simulink model "Ford_T3T6_ArchCnctnDigrm"  (R2016b)
settings: Solver=FixedStepDiscrete  StartTime=0.0  StopTime=10.0  RelTol=1e-3  EnableMultiTasking=on
libraries: canmsglib x15
(part 2 of 15)

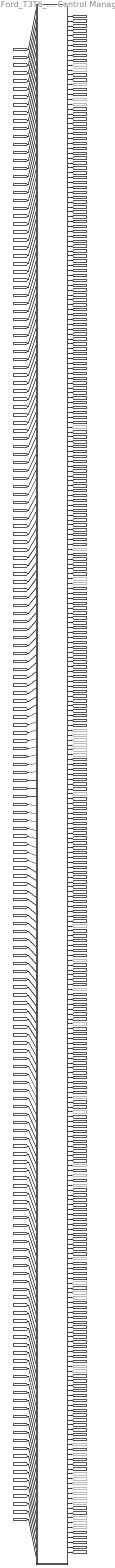
== system Ford_T3T6_ArchCnctnDigrm/Motor Control Manager ==
  AR300FORDA_MotCtrlMgr : Subsystem  Tag=1.0.X  Description=This component handles runnable scheduling of MotorControl and MotorControlx2 runnables. This also defines all of the Motor Control related data and is resposible for the runnables providing the data interface to the RTE.
      settings: AttributesFormatString=Version: %<Tag>
  AR300FORDA_MotCtrlMgr_BattRtnCurrAdc : Goto  Commented=on  GotoTag=BattRtnCurrAdc  TagVisibility=global
  AR300FORDA_MotCtrlMgr_BattRtnCurrAdcFaild : Goto  Commented=on  GotoTag=BattRtnCurrAdcFaild  TagVisibility=global
  AR300FORDA_MotCtrlMgr_BattVltgAdcFaild : Goto  Commented=on  GotoTag=BattVltgAdcFaild  TagVisibility=global
  AR300FORDA_MotCtrlMgr_CurrMeasWrmIninTestCmpl : Goto  Commented=on  GotoTag=CurrMeasWrmIninTestCmpl  TagVisibility=global
  AR300FORDA_MotCtrlMgr_EcuId : Goto  Commented=on  GotoTag=EcuId  TagVisibility=global
  AR300FORDA_MotCtrlMgr_MotBackEmfVltg : Goto  Commented=on  GotoTag=MotBackEmfVltg  TagVisibility=global
  AR300FORDA_MotCtrlMgr_MotCtrlAdc0RawRes : Goto  Commented=on  GotoTag=MotCtrlAdc0RawRes  TagVisibility=global
  AR300FORDA_MotCtrlMgr_MotCtrlAdc0ScanGroup2Ref0 : Goto  Commented=on  GotoTag=MotCtrlAdc0ScanGroup2Ref0  TagVisibility=global
  AR300FORDA_MotCtrlMgr_MotCtrlAdc0ScanGroup2Ref1 : Goto  Commented=on  GotoTag=MotCtrlAdc0ScanGroup2Ref1  TagVisibility=global
  AR300FORDA_MotCtrlMgr_MotCtrlAdc0ScanGroup3Ref0 : Goto  Commented=on  GotoTag=MotCtrlAdc0ScanGroup3Ref0  TagVisibility=global
  AR300FORDA_MotCtrlMgr_MotCtrlAdc0ScanGroup3Ref1 : Goto  Commented=on  GotoTag=MotCtrlAdc0ScanGroup3Ref1  TagVisibility=global
  AR300FORDA_MotCtrlMgr_MotCtrlAdc1RawRes : Goto  Commented=on  GotoTag=MotCtrlAdc1RawRes  TagVisibility=global
  AR300FORDA_MotCtrlMgr_MotCtrlCurrMeasMotAgCorrd : Goto  Commented=on  GotoTag=MotCtrlCurrMeasMotAgCorrd  TagVisibility=global
  AR300FORDA_MotCtrlMgr_MotCtrlMotAg5Cos : Goto  Commented=on  GotoTag=MotCtrlMotAg5Cos  TagVisibility=global
  AR300FORDA_MotCtrlMgr_MotCtrlMotAg5Sin : Goto  Commented=on  GotoTag=MotCtrlMotAg5Sin  TagVisibility=global
  AR300FORDA_MotCtrlMgr_MotCtrlMotAg6Cos : Goto  Commented=on  GotoTag=MotCtrlMotAg6Cos  TagVisibility=global
  AR300FORDA_MotCtrlMgr_MotCtrlMotAg6Sin : Goto  Commented=on  GotoTag=MotCtrlMotAg6Sin  TagVisibility=global
  AR300FORDA_MotCtrlMgr_MotCtrlMotAgElec : Goto  Commented=on  GotoTag=MotCtrlMotAgElec  TagVisibility=global
  AR300FORDA_MotCtrlMgr_MotCtrlMotAgMeasTi : Goto  Commented=on  GotoTag=MotCtrlMotAgMeasTi  TagVisibility=global
  AR300FORDA_MotCtrlMgr_MotCtrlMotCurrAdcVlyA : Goto  Commented=on  GotoTag=MotCtrlMotCurrAdcVlyA  TagVisibility=global
  AR300FORDA_MotCtrlMgr_MotCtrlMotCurrAdcVlyB : Goto  Commented=on  GotoTag=MotCtrlMotCurrAdcVlyB  TagVisibility=global
  AR300FORDA_MotCtrlMgr_MotCtrlMotCurrAdcVlyC : Goto  Commented=on  GotoTag=MotCtrlMotCurrAdcVlyC  TagVisibility=global
  AR300FORDA_MotCtrlMgr_MotCtrlMotCurrDax : Goto  Commented=on  GotoTag=MotCtrlMotCurrDax  TagVisibility=global
  AR300FORDA_MotCtrlMgr_MotCtrlMotCurrQax : Goto  Commented=on  GotoTag=MotCtrlMotCurrQax  TagVisibility=global
  AR300FORDA_MotCtrlMgr_MotCtrlMotCurrQaxCoggCmd : Goto  Commented=on  GotoTag=MotCtrlMotCurrQaxCoggCmd  TagVisibility=global
  AR300FORDA_MotCtrlMgr_MotCtrlMotCurrQaxRplCmd : Goto  Commented=on  GotoTag=MotCtrlMotCurrQaxRplCmd  TagVisibility=global
  AR300FORDA_MotCtrlMgr_MotCtrlMotModlnIdx : Goto  Commented=on  GotoTag=MotCtrlMotModlnIdx  TagVisibility=global
  AR300FORDA_MotCtrlMgr_MotCtrlMotPhaAdv : Goto  Commented=on  GotoTag=MotCtrlMotPhaAdv  TagVisibility=global
  AR300FORDA_MotCtrlMgr_MotCtrlMotVltgDax : Goto  Commented=on  GotoTag=MotCtrlMotVltgDax  TagVisibility=global
  AR300FORDA_MotCtrlMgr_MotCtrlMotVltgQax : Goto  Commented=on  GotoTag=MotCtrlMotVltgQax  TagVisibility=global
  AR300FORDA_MotCtrlMgr_MotCtrlPhaOnTiA : Goto  Commented=on  GotoTag=MotCtrlPhaOnTiA  TagVisibility=global
  AR300FORDA_MotCtrlMgr_MotCtrlPhaOnTiB : Goto  Commented=on  GotoTag=MotCtrlPhaOnTiB  TagVisibility=global
  AR300FORDA_MotCtrlMgr_MotCtrlPhaOnTiC : Goto  Commented=on  GotoTag=MotCtrlPhaOnTiC  TagVisibility=global
  AR300FORDA_MotCtrlMgr_MotCtrlPhaOnTiSumA : Goto  Commented=on  GotoTag=MotCtrlPhaOnTiSumA  TagVisibility=global
  AR300FORDA_MotCtrlMgr_MotCtrlPhaOnTiSumB : Goto  Commented=on  GotoTag=MotCtrlPhaOnTiSumB  TagVisibility=global
  AR300FORDA_MotCtrlMgr_MotCtrlPhaOnTiSumC : Goto  Commented=on  GotoTag=MotCtrlPhaOnTiSumC  TagVisibility=global
  AR300FORDA_MotCtrlMgr_MotCtrlPwmPerd : Goto  Commented=on  GotoTag=MotCtrlPwmPerd  TagVisibility=global
  AR300FORDA_MotCtrlMgr_MotCtrlSwCalEna : Goto  Commented=on  GotoTag=MotCtrlSwCalEna  TagVisibility=global
  AR300FORDA_MotCtrlMgr_MotCtrlSwCalModlnIdx : Goto  Commented=on  GotoTag=MotCtrlSwCalModlnIdx  TagVisibility=global
  AR300FORDA_MotCtrlMgr_MotCtrlSwCalPosnIdx : Goto  Commented=on  GotoTag=MotCtrlSwCalPosnIdx  TagVisibility=global
  AR300FORDA_MotCtrlMgr_MotCurrQlfr1 : Goto  Commented=on  GotoTag=MotCurrQlfr1  TagVisibility=global
  AR300FORDA_MotCtrlMgr_MotInduDaxEstimdIvs : Goto  Commented=on  GotoTag=MotInduDaxEstimdIvs  TagVisibility=global
  AR300FORDA_MotCtrlMgr_MotInduQaxEstimdIvs : Goto  Commented=on  GotoTag=MotInduQaxEstimdIvs  TagVisibility=global
  tag scope: Adc0DynRef=global, Adc0RawRes=global, Adc0ScanGroup2Ref0=global, Adc0ScanGroup2Ref1=global, Adc0ScanGroup3Ref0=global, Adc0ScanGroup3Ref1=global, Adc0SelfDiag0=global, Adc0SelfDiag2=global, Adc0SelfDiag4=global, Adc1RawRes=global, BattRtnCurrAmprFastLoop=global, BattVltgAdc=global, CmuOffs=global, CurrMeasMotAgCorrd=global, FastLoopCntr=global, HwTq0Idx=global, HwTq0MissErrCntr=global, HwTq0SentComSts=global, HwTq0SentData=global, HwTq2Idx=global, HwTq2MissErrCntr=global, HwTq2SentComSts=global, HwTq2SentData=global, HwTq4Buf=global, HwTq4RawAdc=global, HwTq4RawAdcFaild=global, HwTq4RawFastAdc=global, HwTq4RawFastAdcBuf=global, HwTq5Buf=global, HwTq5RawAdc=global, HwTq5RawAdcFaild=global, HwTq5RawFastAdc=global, HwTq5RawFastAdcBuf=global, HwTq8Idx=global, HwTq8MissErrCntr=global, HwTq8SentComSts=global, HwTq8SentData=global, MotAg0ErrReg=global, MotAg0Mecl=global, MotAg0MeclRollgCntr=global, MotAg0ParFltCnt=global, MotAg0RawMecl=global, MotAg0RawRes=global, MotAg0SpiMecl=global, MotAg0TurnCntrReg=global, MotAg0VltgFltCnt=global, MotAg0WarnReg=global, MotAg1ErrReg=global, MotAg1Mecl=global, MotAg1MeclRollgCntr=global, MotAg1ParFltCnt=global, MotAg1RawMecl=global, MotAg1RawRes=global, MotAg1SpiMecl=global, MotAg1TurnCntrReg=global, MotAg1VltgFltCnt=global, MotAg1WarnReg=global, MotAg3Mecl=global, MotAg4Mecl=global, MotAg5Cos=global, MotAg5MeasTi=global, MotAg5Mecl=global, MotAg5RawMecl=global, MotAg5Sin=global, MotAg6Cos=global, MotAg6MeasTi=global, MotAg6Mecl=global, MotAg6RawMecl=global, MotAg6Sin=global, MotAgBuf=global, MotAgBufIdx=global, MotAgBuf_SigOut=global, MotAgCumvAlgndMrfRev=global, MotAgCumvInid=global, MotAgElec=global, MotAgMeasTi=global, MotAgMecl=global, MotAgTiBuf=global, MotAgTiBuf_SigOut=global, MotCtrlAdcDiagcEndPtrOutp=global, MotCtrlAdcDiagcStrtPtrOutp=global, MotCtrlBattRtnCurrAdc=global, MotCtrlBrdgVltg=global, MotCtrlCtrlrTFild=global, MotCtrlCurrMeasCorrlnSts=global, MotCtrlCurrMeasLoaMtgtnEna=global, MotCtrlCurrMeasWrmIninTestCmpl=global, MotCtrlDiagcStsIvtr1Inactv=global, MotCtrlDiagcStsIvtr2Inactv=global, MotCtrlDualEcuMotCtrlMtgtnEna=global, MotCtrlEcuTFild=global, MotCtrlHwTq4Raw=global, MotCtrlHwTq4RawFastAdc=global, MotCtrlHwTq5Raw=global, MotCtrlHwTq5RawFastAdc=global, MotCtrlIvtrFetFltPha=global, MotCtrlIvtrFetFltTyp=global, MotCtrlIvtrLoaMtgtnEna=global, MotCtrlLoopCntr2MilliSec=global, MotCtrlMfgEnaSt=global, MotCtrlMotAg0ABIFaild=global, MotCtrlMotAg0Offs=global, MotCtrlMotAg0QepFaild=global, MotCtrlMotAg0RawRes=global, MotCtrlMotAg1ABIFaild=global, MotCtrlMotAg1Offs=global, MotCtrlMotAg1QepFaild=global, MotCtrlMotAg1RawRes=global, MotCtrlMotAg2Cos=global, MotCtrlMotAg2CosAdcFaild=global, MotCtrlMotAg2Sin=global, MotCtrlMotAg2SinAdcFaild=global, MotCtrlMotAg5CosAdcFaild=global, MotCtrlMotAg5CosRtAmpRecpr1=global, MotCtrlMotAg5CosRtAmpRecpr=global, MotCtrlMotAg5CosRtOffs1=global, MotCtrlMotAg5CosRtOffs=global, MotCtrlMotAg5Polarity=global, MotCtrlMotAg5SinAdcFaild=global, MotCtrlMotAg5SinRtAmpRecpr1=global, MotCtrlMotAg5SinRtAmpRecpr=global, MotCtrlMotAg5SinRtOffs1=global, MotCtrlMotAg5SinRtOffs=global, MotCtrlMotAg6CosAdcFaild=global, MotCtrlMotAg6CosRtAmpRecpr1=global, MotCtrlMotAg6CosRtAmpRecpr=global, MotCtrlMotAg6CosRtOffs1=global, MotCtrlMotAg6CosRtOffs=global, MotCtrlMotAg6Polarity=global, MotCtrlMotAg6SinAdcFaild=global, MotCtrlMotAg6SinRtAmpRecpr1=global, MotCtrlMotAg6SinRtAmpRecpr=global, MotCtrlMotAg6SinRtOffs1=global, MotCtrlMotAg6SinRtOffs=global, MotCtrlMotAgAMecl=global, MotCtrlMotAgAMeclQlfr=global, MotCtrlMotAgAMeclRollgCntr=global, MotCtrlMotAgBMecl=global, MotCtrlMotAgBMeclQlfr=global, MotCtrlMotAgBMeclRollgCntr=global, MotCtrlMotAgBuf=global, MotCtrlMotAgBuf_SigIn=global, MotCtrlMotAgCorrd=global, MotCtrlMotAgElecDly=global, MotCtrlMotAgElecDlyRpl=global, MotCtrlMotAgMecl0Polarity=global, MotCtrlMotAgMecl1Polarity=global, MotCtrlMotAgMecl=global, MotCtrlMotAgMeclCorrlnSt=global, MotCtrlMotAgMeclCorrlnSts=global, MotCtrlMotAgTiBuf=global, MotCtrlMotAgTiBuf_SigIn=global, MotCtrlMotAndThermProtnLoaMod=global, MotCtrlMotBackEmfVltg=global, MotCtrlMotCurr=global, MotCtrlMotCurrAdcVlyAAdcFaild=global, MotCtrlMotCurrAdcVlyBAdcFaild=global, MotCtrlMotCurrAdcVlyCAdcFaild=global, MotCtrlMotCurrAdcVlyD=global, MotCtrlMotCurrAdcVlyDAdcFaild=global, MotCtrlMotCurrAdcVlyE=global, MotCtrlMotCurrAdcVlyEAdcFaild=global, MotCtrlMotCurrAdcVlyF=global, MotCtrlMotCurrAdcVlyFAdcFaild=global, MotCtrlMotCurrCmd=global, MotCtrlMotCurrCorrdA=global, MotCtrlMotCurrCorrdB=global, MotCtrlMotCurrCorrdC=global, MotCtrlMotCurrCorrdD=global, MotCtrlMotCurrCorrdE=global, MotCtrlMotCurrCorrdF=global, MotCtrlMotCurrDaxCmd=global, MotCtrlMotCurrDaxMax=global, MotCtrlMotCurrEolCalSt=global, MotCtrlMotCurrLoaMtgtnEna=global, MotCtrlMotCurrQaxCmd=global, MotCtrlMotCurrQaxToMotTqGain=global, MotCtrlMotCurrQlfr1=global, MotCtrlMotCurrQlfr2=global, MotCtrlMotCurrRollgCntr1=global, MotCtrlMotCurrRollgCntr2=global, MotCtrlMotDampgDax=global, MotCtrlMotDampgQax=global, MotCtrlMotElecMeclPolarity=global, MotCtrlMotInduDaxEstimdIvs=global, MotCtrlMotInduQaxEstimdIvs=global, MotCtrlMotIntglGain=global, MotCtrlMotIntglGainDax=global, MotCtrlMotIntglGainQax=global, MotCtrlMotPropGain=global, MotCtrlMotPropGainDax=global, MotCtrlMotPropGainQax=global, MotCtrlMotREstimd=global, MotCtrlMotReacncDax=global, MotCtrlMotReacncQax=global, MotCtrlMotTqRplCoggOrder1Mgn=global, MotCtrlMotTqRplCoggOrder1Pha=global, MotCtrlMotTqRplCoggOrder2Mgn=global, MotCtrlMotTqRplCoggOrder2Pha=global, MotCtrlMotTqRplCoggOrder3Mgn=global, MotCtrlMotTqRplCoggOrder3Pha=global, MotCtrlMotVelMrf=global, MotCtrlMotVltgCmdPolarity=global, MotCtrlMotVltgDaxFf=global, MotCtrlMotVltgQaxFf=global, MotCtrlPhaDiscnctDiagcActv=global, MotCtrlPhaDiscnctDiagcPwmVect=global, MotCtrlSampleRdyFlgInp=global, MotCtrlStrtUpSt=global, MotCtrlSysSt=global, MotCtrlTSG31CMPVE=global, MotCtrlTSG31CMPWE=global, MotCtrlTSG31DCMP0E=global, MotCtrlVehSpd=global, MotCurr=global, MotCurrAdcPeakA=global, MotCurrAdcPeakB=global, MotCurrAdcPeakC=global, MotCurrAdcPeakD=global, MotCurrAdcPeakE=global, MotCurrAdcPeakF=global, MotCurrAdcVlyA=global, MotCurrAdcVlyB=global, MotCurrAdcVlyC=global, MotCurrAdcVlyD=global, MotCurrAdcVlyE=global, MotCurrAdcVlyF=global, MotCurrCorrdA=global, MotCurrCorrdB=global, MotCurrCorrdC=global, MotCurrCorrdD=global, MotCurrCorrdE=global, MotCurrCorrdF=global, MotCurrDax=global, MotCurrQax=global, MotCurrQaxCmdFinal=global, MotCurrQaxCoggCmd=global, MotCurrQaxRplCmd=global, MotCurrQlfr2=global, MotCurrRollgCntr1=global, MotCurrRollgCntr2=global, MotCurrSnsrOffs1=global, MotCurrSnsrOffs2=global, MotModlnIdx=global, MotPhaAdv=global, MotVltg=global, MotVltgCmdPolarity=global, MotVltgDax=global, MotVltgDaxFild=global, MotVltgQax=global, MotVltgQaxFild=global, Ntc5DErrCnt=global, Ntc6DErrCnt=global, PhaOnTiA=global, PhaOnTiB=global, PhaOnTiC=global, PhaOnTiSumA=global, PhaOnTiSumB=global, PhaOnTiSumC=global, PwmPerd=global, RegOutpCSIH1RRA=global, SampleRdyFlgOutp=global, SlowLoopCntr=global, SwCalEna=global, SwCalModlnIdx=global, SwCalPosnIdx=global, TSG31CMP0E=global, TSG31CMP12E=global, TSG31CMPUE=global, TSG31CMPVE=global, TSG31CMPWE=global, TSG31DCMP0E=global
  wires:
  [AdcDiagcEndPtrOutp] -> AR300FORDA_MotCtrlMgr/1(AdcDiagcEndPtrOutp)
  [AdcDiagcStrtPtrOutp] -> AR300FORDA_MotCtrlMgr/2(AdcDiagcStrtPtrOutp)
  [BrdgVltg] -> AR300FORDA_MotCtrlMgr/3(BrdgVltg)
  [CtrlrTFild] -> AR300FORDA_MotCtrlMgr/4(CtrlrTFild)
  [CurrMeasCorrlnSts] -> AR300FORDA_MotCtrlMgr/5(CurrMeasCorrlnSts)
  [CurrMeasLoaMtgtnEna] -> AR300FORDA_MotCtrlMgr/6(CurrMeasLoaMtgtnEna)
  [DiagcStsIvtr1Inactv] -> AR300FORDA_MotCtrlMgr/7(DiagcStsIvtr1Inactv)
  [DiagcStsIvtr2Inactv] -> AR300FORDA_MotCtrlMgr/8(DiagcStsIvtr2Inactv)
  [DualEcuMotCtrlMtgtnEna] -> AR300FORDA_MotCtrlMgr/9(DualEcuMotCtrlMtgtnEna)
  [EcuTFild] -> AR300FORDA_MotCtrlMgr/10(EcuTFild)
  [HwTq4Raw] -> AR300FORDA_MotCtrlMgr/11(HwTq4Raw)
  [HwTq5Raw] -> AR300FORDA_MotCtrlMgr/12(HwTq5Raw)
  [IvtrFetFltPha] -> AR300FORDA_MotCtrlMgr/13(IvtrFetFltPha)
  [IvtrFetFltTyp] -> AR300FORDA_MotCtrlMgr/14(IvtrFetFltTyp)
  [IvtrLoaMtgtnEna] -> AR300FORDA_MotCtrlMgr/15(IvtrLoaMtgtnEna)
  [LoopCntr2MilliSec] -> AR300FORDA_MotCtrlMgr/16(LoopCntr2MilliSec)
  [MfgEnaSt] -> AR300FORDA_MotCtrlMgr/17(MfgEnaSt)
  [MotAg0ABIFaild] -> AR300FORDA_MotCtrlMgr/18(MotAg0ABIFaild)
  [MotAg0Offs] -> AR300FORDA_MotCtrlMgr/19(MotAg0Offs)
  [MotAg0QepFaild] -> AR300FORDA_MotCtrlMgr/20(MotAg0QepFaild)
  [MotAg1ABIFaild] -> AR300FORDA_MotCtrlMgr/21(MotAg1ABIFaild)
  [MotAg1Offs] -> AR300FORDA_MotCtrlMgr/22(MotAg1Offs)
  [MotAg1QepFaild] -> AR300FORDA_MotCtrlMgr/23(MotAg1QepFaild)
  [MotAg2Cos] -> AR300FORDA_MotCtrlMgr/24(MotAg2Cos)
  [MotAg2CosAdcFaild] -> AR300FORDA_MotCtrlMgr/25(MotAg2CosAdcFaild)
  [MotAg2Sin] -> AR300FORDA_MotCtrlMgr/26(MotAg2Sin)
  [MotAg2SinAdcFaild] -> AR300FORDA_MotCtrlMgr/27(MotAg2SinAdcFaild)
  [MotAg5CosAdcFaild] -> AR300FORDA_MotCtrlMgr/28(MotAg5CosAdcFaild)
  [MotAg5CosRtAmpRecpr] -> AR300FORDA_MotCtrlMgr/29(MotAg5CosRtAmpRecpr)
  [MotAg5CosRtAmpRecpr1] -> AR300FORDA_MotCtrlMgr/30(MotAg5CosRtAmpRecpr1)
  [MotAg5CosRtOffs] -> AR300FORDA_MotCtrlMgr/31(MotAg5CosRtOffs)
  [MotAg5CosRtOffs1] -> AR300FORDA_MotCtrlMgr/32(MotAg5CosRtOffs1)
  [MotAg5Polarity] -> AR300FORDA_MotCtrlMgr/33(MotAg5Polarity)
  [MotAg5SinAdcFaild] -> AR300FORDA_MotCtrlMgr/34(MotAg5SinAdcFaild)
  [MotAg5SinRtAmpRecpr] -> AR300FORDA_MotCtrlMgr/35(MotAg5SinRtAmpRecpr)
  [MotAg5SinRtAmpRecpr1] -> AR300FORDA_MotCtrlMgr/36(MotAg5SinRtAmpRecpr1)
  [MotAg5SinRtOffs] -> AR300FORDA_MotCtrlMgr/37(MotAg5SinRtOffs)
  [MotAg5SinRtOffs1] -> AR300FORDA_MotCtrlMgr/38(MotAg5SinRtOffs1)
  [MotAg6CosAdcFaild] -> AR300FORDA_MotCtrlMgr/39(MotAg6CosAdcFaild)
  [MotAg6CosRtAmpRecpr] -> AR300FORDA_MotCtrlMgr/40(MotAg6CosRtAmpRecpr)
  [MotAg6CosRtAmpRecpr1] -> AR300FORDA_MotCtrlMgr/41(MotAg6CosRtAmpRecpr1)
  [MotAg6CosRtOffs] -> AR300FORDA_MotCtrlMgr/42(MotAg6CosRtOffs)
  [MotAg6CosRtOffs1] -> AR300FORDA_MotCtrlMgr/43(MotAg6CosRtOffs1)
  [MotAg6Polarity] -> AR300FORDA_MotCtrlMgr/44(MotAg6Polarity)
  [MotAg6SinAdcFaild] -> AR300FORDA_MotCtrlMgr/45(MotAg6SinAdcFaild)
  [MotAg6SinRtAmpRecpr] -> AR300FORDA_MotCtrlMgr/46(MotAg6SinRtAmpRecpr)
  [MotAg6SinRtAmpRecpr1] -> AR300FORDA_MotCtrlMgr/47(MotAg6SinRtAmpRecpr1)
  [MotAg6SinRtOffs] -> AR300FORDA_MotCtrlMgr/48(MotAg6SinRtOffs)
  [MotAg6SinRtOffs1] -> AR300FORDA_MotCtrlMgr/49(MotAg6SinRtOffs1)
  [MotAgAMecl] -> AR300FORDA_MotCtrlMgr/50(MotAgAMecl)
  [MotAgAMeclQlfr] -> AR300FORDA_MotCtrlMgr/51(MotAgAMeclQlfr)
  [MotAgAMeclRollgCntr] -> AR300FORDA_MotCtrlMgr/52(MotAgAMeclRollgCntr)
  [MotAgBMecl] -> AR300FORDA_MotCtrlMgr/53(MotAgBMecl)
  [MotAgBMeclQlfr] -> AR300FORDA_MotCtrlMgr/54(MotAgBMeclQlfr)
  [MotAgBMeclRollgCntr] -> AR300FORDA_MotCtrlMgr/55(MotAgBMeclRollgCntr)
  [MotAgBuf_SigIn] -> AR300FORDA_MotCtrlMgr/56(MotAgBuf_SigIn)
  [MotAgCorrd] -> AR300FORDA_MotCtrlMgr/57(MotAgCorrd)
  [MotAgElecDly] -> AR300FORDA_MotCtrlMgr/58(MotAgElecDly)
  [MotAgElecDlyRpl] -> AR300FORDA_MotCtrlMgr/59(MotAgElecDlyRpl)
  [MotAgMecl0Polarity] -> AR300FORDA_MotCtrlMgr/60(MotAgMecl0Polarity)
  [MotAgMecl1Polarity] -> AR300FORDA_MotCtrlMgr/61(MotAgMecl1Polarity)
  [MotAgMeclCorrlnSt] -> AR300FORDA_MotCtrlMgr/62(MotAgMeclCorrlnSt)
  [MotAgMeclCorrlnSts] -> AR300FORDA_MotCtrlMgr/63(MotAgMeclCorrlnSts)
  [MotAgTiBuf_SigIn] -> AR300FORDA_MotCtrlMgr/64(MotAgTiBuf_SigIn)
  [MotAndThermProtnLoaMod] -> AR300FORDA_MotCtrlMgr/65(MotAndThermProtnLoaMod)
  [MotCurrAdcVlyAAdcFaild] -> AR300FORDA_MotCtrlMgr/66(MotCurrAdcVlyAAdcFaild)
  [MotCurrAdcVlyBAdcFaild] -> AR300FORDA_MotCtrlMgr/67(MotCurrAdcVlyBAdcFaild)
  [MotCurrAdcVlyCAdcFaild] -> AR300FORDA_MotCtrlMgr/68(MotCurrAdcVlyCAdcFaild)
  [MotCurrAdcVlyDAdcFaild] -> AR300FORDA_MotCtrlMgr/69(MotCurrAdcVlyDAdcFaild)
  [MotCurrAdcVlyEAdcFaild] -> AR300FORDA_MotCtrlMgr/70(MotCurrAdcVlyEAdcFaild)
  [MotCurrAdcVlyFAdcFaild] -> AR300FORDA_MotCtrlMgr/71(MotCurrAdcVlyFAdcFaild)
  [MotCurrCmd] -> AR300FORDA_MotCtrlMgr/72(MotCurrCmd)
  [MotCurrDaxCmd] -> AR300FORDA_MotCtrlMgr/73(MotCurrDaxCmd)
  [MotCurrDaxMax] -> AR300FORDA_MotCtrlMgr/74(MotCurrDaxMax)
  [MotCurrEolCalSt] -> AR300FORDA_MotCtrlMgr/75(MotCurrEolCalSt)
  [MotCurrLoaMtgtnEna] -> AR300FORDA_MotCtrlMgr/76(MotCurrLoaMtgtnEna)
  [MotCurrQaxCmd] -> AR300FORDA_MotCtrlMgr/77(MotCurrQaxCmd)
  [MotCurrQaxToMotTqGain] -> AR300FORDA_MotCtrlMgr/78(MotCurrQaxToMotTqGain)
  [MotDampgDax] -> AR300FORDA_MotCtrlMgr/79(MotDampgDax)
  [MotDampgQax] -> AR300FORDA_MotCtrlMgr/80(MotDampgQax)
  [MotElecMeclPolarity] -> AR300FORDA_MotCtrlMgr/81(MotElecMeclPolarity)
  [MotIntglGain] -> AR300FORDA_MotCtrlMgr/82(MotIntglGain)
  [MotIntglGainDax] -> AR300FORDA_MotCtrlMgr/83(MotIntglGainDax)
  [MotIntglGainQax] -> AR300FORDA_MotCtrlMgr/84(MotIntglGainQax)
  [MotPropGain] -> AR300FORDA_MotCtrlMgr/85(MotPropGain)
  [MotPropGainDax] -> AR300FORDA_MotCtrlMgr/86(MotPropGainDax)
  [MotPropGainQax] -> AR300FORDA_MotCtrlMgr/87(MotPropGainQax)
  [MotREstimd] -> AR300FORDA_MotCtrlMgr/88(MotREstimd)
  [MotReacncDax] -> AR300FORDA_MotCtrlMgr/89(MotReacncDax)
  [MotReacncQax] -> AR300FORDA_MotCtrlMgr/90(MotReacncQax)
  [MotTqRplCoggOrder1Mgn] -> AR300FORDA_MotCtrlMgr/91(MotTqRplCoggOrder1Mgn)
  [MotTqRplCoggOrder1Pha] -> AR300FORDA_MotCtrlMgr/92(MotTqRplCoggOrder1Pha)
  [MotTqRplCoggOrder2Mgn] -> AR300FORDA_MotCtrlMgr/93(MotTqRplCoggOrder2Mgn)
  [MotTqRplCoggOrder2Pha] -> AR300FORDA_MotCtrlMgr/94(MotTqRplCoggOrder2Pha)
  [MotTqRplCoggOrder3Mgn] -> AR300FORDA_MotCtrlMgr/95(MotTqRplCoggOrder3Mgn)
  [MotTqRplCoggOrder3Pha] -> AR300FORDA_MotCtrlMgr/96(MotTqRplCoggOrder3Pha)
  [MotVelMrf] -> AR300FORDA_MotCtrlMgr/97(MotVelMrf)
  [MotVltgDaxFf] -> AR300FORDA_MotCtrlMgr/98(MotVltgDaxFf)
  [MotVltgQaxFf] -> AR300FORDA_MotCtrlMgr/99(MotVltgQaxFf)
  [PhaDiscnctDiagcActv] -> AR300FORDA_MotCtrlMgr/100(PhaDiscnctDiagcActv)
  [PhaDiscnctDiagcPwmVect] -> AR300FORDA_MotCtrlMgr/101(PhaDiscnctDiagcPwmVect)
  [SampleRdyFlgInp] -> AR300FORDA_MotCtrlMgr/102(SampleRdyFlgInp)
  [StrtUpSt] -> AR300FORDA_MotCtrlMgr/103(StrtUpSt)
  [SysSt] -> AR300FORDA_MotCtrlMgr/104(SysSt)
  [VehSpd] -> AR300FORDA_MotCtrlMgr/105(VehSpd)
  [MotCtrlAdc0DynRef] -> AR300FORDA_MotCtrlMgr/106(MotCtrlAdc0DynRef)
  [MotCtrlAdc0SelfDiag0] -> AR300FORDA_MotCtrlMgr/107(MotCtrlAdc0SelfDiag0)
  [MotCtrlAdc0SelfDiag2] -> AR300FORDA_MotCtrlMgr/108(MotCtrlAdc0SelfDiag2)
  [MotCtrlAdc0SelfDiag4] -> AR300FORDA_MotCtrlMgr/109(MotCtrlAdc0SelfDiag4)
  [MotCtrlBattRtnCurrAdcFaild] -> AR300FORDA_MotCtrlMgr/110(MotCtrlBattRtnCurrAdcFaild)
  [MotCtrlBattRtnCurrAmprFastLoop] -> AR300FORDA_MotCtrlMgr/111(MotCtrlBattRtnCurrAmprFastLoop)
  [MotCtrlBattVltgAdc] -> AR300FORDA_MotCtrlMgr/112(MotCtrlBattVltgAdc)
  [MotCtrlBattVltgAdcFaild] -> AR300FORDA_MotCtrlMgr/113(MotCtrlBattVltgAdcFaild)
  [MotCtrlCmuOffs] -> AR300FORDA_MotCtrlMgr/114(MotCtrlCmuOffs)
  [MotCtrlFastLoopCntr] -> AR300FORDA_MotCtrlMgr/115(MotCtrlFastLoopCntr)
  [MotCtrlHwTq0Idx] -> AR300FORDA_MotCtrlMgr/116(MotCtrlHwTq0Idx)
  [MotCtrlHwTq0MissErrCntr] -> AR300FORDA_MotCtrlMgr/117(MotCtrlHwTq0MissErrCntr)
  [MotCtrlHwTq0SentComSts] -> AR300FORDA_MotCtrlMgr/118(MotCtrlHwTq0SentComSts)
  [MotCtrlHwTq0SentData] -> AR300FORDA_MotCtrlMgr/119(MotCtrlHwTq0SentData)
  [MotCtrlHwTq2Idx] -> AR300FORDA_MotCtrlMgr/120(MotCtrlHwTq2Idx)
  [MotCtrlHwTq2MissErrCntr] -> AR300FORDA_MotCtrlMgr/121(MotCtrlHwTq2MissErrCntr)
  [MotCtrlHwTq2SentComSts] -> AR300FORDA_MotCtrlMgr/122(MotCtrlHwTq2SentComSts)
  [MotCtrlHwTq2SentData] -> AR300FORDA_MotCtrlMgr/123(MotCtrlHwTq2SentData)
  [MotCtrlHwTq4Buf] -> AR300FORDA_MotCtrlMgr/124(MotCtrlHwTq4Buf)
  [MotCtrlHwTq4RawAdc] -> AR300FORDA_MotCtrlMgr/125(MotCtrlHwTq4RawAdc)
  [MotCtrlHwTq4RawAdcFaild] -> AR300FORDA_MotCtrlMgr/126(MotCtrlHwTq4RawAdcFaild)
  [MotCtrlHwTq4RawFastAdcBuf] -> AR300FORDA_MotCtrlMgr/127(MotCtrlHwTq4RawFastAdcBuf)
  [MotCtrlHwTq5Buf] -> AR300FORDA_MotCtrlMgr/128(MotCtrlHwTq5Buf)
  [MotCtrlHwTq5RawAdc] -> AR300FORDA_MotCtrlMgr/129(MotCtrlHwTq5RawAdc)
  [MotCtrlHwTq5RawAdcFaild] -> AR300FORDA_MotCtrlMgr/130(MotCtrlHwTq5RawAdcFaild)
  [MotCtrlHwTq5RawFastAdcBuf] -> AR300FORDA_MotCtrlMgr/131(MotCtrlHwTq5RawFastAdcBuf)
  [MotCtrlHwTq8Idx] -> AR300FORDA_MotCtrlMgr/132(MotCtrlHwTq8Idx)
  [MotCtrlHwTq8MissErrCntr] -> AR300FORDA_MotCtrlMgr/133(MotCtrlHwTq8MissErrCntr)
  [MotCtrlHwTq8SentComSts] -> AR300FORDA_MotCtrlMgr/134(MotCtrlHwTq8SentComSts)
  [MotCtrlHwTq8SentData] -> AR300FORDA_MotCtrlMgr/135(MotCtrlHwTq8SentData)
  [MotCtrlMotAg0ErrReg] -> AR300FORDA_MotCtrlMgr/136(MotCtrlMotAg0ErrReg)
  [MotCtrlMotAg0Mecl] -> AR300FORDA_MotCtrlMgr/137(MotCtrlMotAg0Mecl)
  [MotCtrlMotAg0MeclRollgCntr] -> AR300FORDA_MotCtrlMgr/138(MotCtrlMotAg0MeclRollgCntr)
  [MotCtrlMotAg0ParFltCnt] -> AR300FORDA_MotCtrlMgr/139(MotCtrlMotAg0ParFltCnt)
  [MotCtrlMotAg0RawMecl] -> AR300FORDA_MotCtrlMgr/140(MotCtrlMotAg0RawMecl)
  [MotCtrlMotAg0SpiMecl] -> AR300FORDA_MotCtrlMgr/141(MotCtrlMotAg0SpiMecl)
  [MotCtrlMotAg0TurnCntrReg] -> AR300FORDA_MotCtrlMgr/142(MotCtrlMotAg0TurnCntrReg)
  [MotCtrlMotAg0VltgFltCnt] -> AR300FORDA_MotCtrlMgr/143(MotCtrlMotAg0VltgFltCnt)
  [MotCtrlMotAg0WarnReg] -> AR300FORDA_MotCtrlMgr/144(MotCtrlMotAg0WarnReg)
  [MotCtrlMotAg1ErrReg] -> AR300FORDA_MotCtrlMgr/145(MotCtrlMotAg1ErrReg)
  [MotCtrlMotAg1Mecl] -> AR300FORDA_MotCtrlMgr/146(MotCtrlMotAg1Mecl)
  [MotCtrlMotAg1MeclRollgCntr] -> AR300FORDA_MotCtrlMgr/147(MotCtrlMotAg1MeclRollgCntr)
  [MotCtrlMotAg1ParFltCnt] -> AR300FORDA_MotCtrlMgr/148(MotCtrlMotAg1ParFltCnt)
  [MotCtrlMotAg1RawMecl] -> AR300FORDA_MotCtrlMgr/149(MotCtrlMotAg1RawMecl)
  [MotCtrlMotAg1SpiMecl] -> AR300FORDA_MotCtrlMgr/150(MotCtrlMotAg1SpiMecl)
  [MotCtrlMotAg1TurnCntrReg] -> AR300FORDA_MotCtrlMgr/151(MotCtrlMotAg1TurnCntrReg)
  [MotCtrlMotAg1VltgFltCnt] -> AR300FORDA_MotCtrlMgr/152(MotCtrlMotAg1VltgFltCnt)
  [MotCtrlMotAg1WarnReg] -> AR300FORDA_MotCtrlMgr/153(MotCtrlMotAg1WarnReg)
  [MotCtrlMotAg3Mecl] -> AR300FORDA_MotCtrlMgr/154(MotCtrlMotAg3Mecl)
  [MotCtrlMotAg4Mecl] -> AR300FORDA_MotCtrlMgr/155(MotCtrlMotAg4Mecl)
  [MotCtrlMotAg5MeasTi] -> AR300FORDA_MotCtrlMgr/156(MotCtrlMotAg5MeasTi)
  [MotCtrlMotAg5Mecl] -> AR300FORDA_MotCtrlMgr/157(MotCtrlMotAg5Mecl)
  [MotCtrlMotAg5RawMecl] -> AR300FORDA_MotCtrlMgr/158(MotCtrlMotAg5RawMecl)
  [MotCtrlMotAg6MeasTi] -> AR300FORDA_MotCtrlMgr/159(MotCtrlMotAg6MeasTi)
  [MotCtrlMotAg6Mecl] -> AR300FORDA_MotCtrlMgr/160(MotCtrlMotAg6Mecl)
  [MotCtrlMotAg6RawMecl] -> AR300FORDA_MotCtrlMgr/161(MotCtrlMotAg6RawMecl)
  [MotCtrlMotAgBufIdx] -> AR300FORDA_MotCtrlMgr/162(MotCtrlMotAgBufIdx)
  [MotCtrlMotAgBuf_SigOut] -> AR300FORDA_MotCtrlMgr/163(MotCtrlMotAgBuf_SigOut)
  [MotCtrlMotAgCumvAlgndMrfRev] -> AR300FORDA_MotCtrlMgr/164(MotCtrlMotAgCumvAlgndMrfRev)
  [MotCtrlMotAgCumvInid] -> AR300FORDA_MotCtrlMgr/165(MotCtrlMotAgCumvInid)
  [MotCtrlMotAgTiBuf_SigOut] -> AR300FORDA_MotCtrlMgr/166(MotCtrlMotAgTiBuf_SigOut)
  [MotCtrlMotCurrAdcPeakA] -> AR300FORDA_MotCtrlMgr/167(MotCtrlMotCurrAdcPeakA)
  [MotCtrlMotCurrAdcPeakB] -> AR300FORDA_MotCtrlMgr/168(MotCtrlMotCurrAdcPeakB)
  [MotCtrlMotCurrAdcPeakC] -> AR300FORDA_MotCtrlMgr/169(MotCtrlMotCurrAdcPeakC)
  [MotCtrlMotCurrAdcPeakD] -> AR300FORDA_MotCtrlMgr/170(MotCtrlMotCurrAdcPeakD)
  [MotCtrlMotCurrAdcPeakE] -> AR300FORDA_MotCtrlMgr/171(MotCtrlMotCurrAdcPeakE)
  [MotCtrlMotCurrAdcPeakF] -> AR300FORDA_MotCtrlMgr/172(MotCtrlMotCurrAdcPeakF)
  [MotCtrlMotCurrQaxCmdFinal] -> AR300FORDA_MotCtrlMgr/173(MotCtrlMotCurrQaxCmdFinal)
  [MotCtrlMotCurrSnsrOffs1] -> AR300FORDA_MotCtrlMgr/174(MotCtrlMotCurrSnsrOffs1)
  [MotCtrlMotCurrSnsrOffs2] -> AR300FORDA_MotCtrlMgr/175(MotCtrlMotCurrSnsrOffs2)
  [MotCtrlMotVltg] -> AR300FORDA_MotCtrlMgr/176(MotCtrlMotVltg)
  [MotCtrlMotVltgDaxFild] -> AR300FORDA_MotCtrlMgr/177(MotCtrlMotVltgDaxFild)
  [MotCtrlMotVltgQaxFild] -> AR300FORDA_MotCtrlMgr/178(MotCtrlMotVltgQaxFild)
  [MotCtrlNtc5DErrCnt] -> AR300FORDA_MotCtrlMgr/179(MotCtrlNtc5DErrCnt)
  [MotCtrlNtc6DErrCnt] -> AR300FORDA_MotCtrlMgr/180(MotCtrlNtc6DErrCnt)
  [MotCtrlRegOutpCSIH1RRA] -> AR300FORDA_MotCtrlMgr/181(MotCtrlRegOutpCSIH1RRA)
  [MotCtrlSampleRdyFlgOutp] -> AR300FORDA_MotCtrlMgr/182(MotCtrlSampleRdyFlgOutp)
  [MotCtrlSlowLoopCntr] -> AR300FORDA_MotCtrlMgr/183(MotCtrlSlowLoopCntr)
  [MotCtrlTSG31CMP0E] -> AR300FORDA_MotCtrlMgr/184(MotCtrlTSG31CMP0E)
  [MotCtrlTSG31CMP12E] -> AR300FORDA_MotCtrlMgr/185(MotCtrlTSG31CMP12E)
  [MotCtrlTSG31CMPUE] -> AR300FORDA_MotCtrlMgr/186(MotCtrlTSG31CMPUE)
  AR300FORDA_MotCtrlMgr/1(Adc0DynRef) -> [Adc0DynRef]
  AR300FORDA_MotCtrlMgr/2(Adc0RawRes) -> [Adc0RawRes]
  AR300FORDA_MotCtrlMgr/3(Adc0ScanGroup2Ref0) -> [Adc0ScanGroup2Ref0]
  AR300FORDA_MotCtrlMgr/4(Adc0ScanGroup2Ref1) -> [Adc0ScanGroup2Ref1]
  AR300FORDA_MotCtrlMgr/5(Adc0ScanGroup3Ref0) -> [Adc0ScanGroup3Ref0]
  AR300FORDA_MotCtrlMgr/6(Adc0ScanGroup3Ref1) -> [Adc0ScanGroup3Ref1]
  AR300FORDA_MotCtrlMgr/7(Adc0SelfDiag0) -> [Adc0SelfDiag0]
  AR300FORDA_MotCtrlMgr/8(Adc0SelfDiag2) -> [Adc0SelfDiag2]
  AR300FORDA_MotCtrlMgr/9(Adc0SelfDiag4) -> [Adc0SelfDiag4]
  AR300FORDA_MotCtrlMgr/10(Adc1RawRes) -> [Adc1RawRes]
  AR300FORDA_MotCtrlMgr/11(BattRtnCurrAdc) -> AR300FORDA_MotCtrlMgr_BattRtnCurrAdc/1
  AR300FORDA_MotCtrlMgr/12(BattRtnCurrAdcFaild) -> AR300FORDA_MotCtrlMgr_BattRtnCurrAdcFaild/1
  AR300FORDA_MotCtrlMgr/13(BattRtnCurrAmprFastLoop) -> [BattRtnCurrAmprFastLoop]
  AR300FORDA_MotCtrlMgr/14(BattVltgAdc) -> [BattVltgAdc]
  AR300FORDA_MotCtrlMgr/15(BattVltgAdcFaild) -> AR300FORDA_MotCtrlMgr_BattVltgAdcFaild/1
  AR300FORDA_MotCtrlMgr/16(CmuOffs) -> [CmuOffs]
  AR300FORDA_MotCtrlMgr/17(CurrMeasMotAgCorrd) -> [CurrMeasMotAgCorrd]
  AR300FORDA_MotCtrlMgr/18(CurrMeasWrmIninTestCmpl) -> AR300FORDA_MotCtrlMgr_CurrMeasWrmIninTestCmpl/1
  AR300FORDA_MotCtrlMgr/19(EcuId) -> AR300FORDA_MotCtrlMgr_EcuId/1
  AR300FORDA_MotCtrlMgr/20(FastLoopCntr) -> [FastLoopCntr]
  AR300FORDA_MotCtrlMgr/21(HwTq0Idx) -> [HwTq0Idx]
  AR300FORDA_MotCtrlMgr/22(HwTq0MissErrCntr) -> [HwTq0MissErrCntr]
  AR300FORDA_MotCtrlMgr/23(HwTq0SentComSts) -> [HwTq0SentComSts]
  AR300FORDA_MotCtrlMgr/24(HwTq0SentData) -> [HwTq0SentData]
  AR300FORDA_MotCtrlMgr/25(HwTq2Idx) -> [HwTq2Idx]
  AR300FORDA_MotCtrlMgr/26(HwTq2MissErrCntr) -> [HwTq2MissErrCntr]
  AR300FORDA_MotCtrlMgr/27(HwTq2SentComSts) -> [HwTq2SentComSts]
  AR300FORDA_MotCtrlMgr/28(HwTq2SentData) -> [HwTq2SentData]
  AR300FORDA_MotCtrlMgr/29(HwTq4Buf) -> [HwTq4Buf]
  AR300FORDA_MotCtrlMgr/30(HwTq4RawAdc) -> [HwTq4RawAdc]
  AR300FORDA_MotCtrlMgr/31(HwTq4RawAdcFaild) -> [HwTq4RawAdcFaild]
  AR300FORDA_MotCtrlMgr/32(HwTq4RawFastAdc) -> [HwTq4RawFastAdc]
  AR300FORDA_MotCtrlMgr/33(HwTq4RawFastAdcBuf) -> [HwTq4RawFastAdcBuf]
  AR300FORDA_MotCtrlMgr/34(HwTq5Buf) -> [HwTq5Buf]
  AR300FORDA_MotCtrlMgr/35(HwTq5RawAdc) -> [HwTq5RawAdc]
  AR300FORDA_MotCtrlMgr/36(HwTq5RawAdcFaild) -> [HwTq5RawAdcFaild]
  AR300FORDA_MotCtrlMgr/37(HwTq5RawFastAdc) -> [HwTq5RawFastAdc]
  AR300FORDA_MotCtrlMgr/38(HwTq5RawFastAdcBuf) -> [HwTq5RawFastAdcBuf]
  AR300FORDA_MotCtrlMgr/39(HwTq8Idx) -> [HwTq8Idx]
  AR300FORDA_MotCtrlMgr/40(HwTq8MissErrCntr) -> [HwTq8MissErrCntr]
  AR300FORDA_MotCtrlMgr/41(HwTq8SentComSts) -> [HwTq8SentComSts]
  AR300FORDA_MotCtrlMgr/42(HwTq8SentData) -> [HwTq8SentData]
  AR300FORDA_MotCtrlMgr/43(MotAg0ErrReg) -> [MotAg0ErrReg]
  AR300FORDA_MotCtrlMgr/44(MotAg0Mecl) -> [MotAg0Mecl]
  AR300FORDA_MotCtrlMgr/45(MotAg0MeclRollgCntr) -> [MotAg0MeclRollgCntr]
  AR300FORDA_MotCtrlMgr/46(MotAg0ParFltCnt) -> [MotAg0ParFltCnt]
  AR300FORDA_MotCtrlMgr/47(MotAg0RawMecl) -> [MotAg0RawMecl]
  AR300FORDA_MotCtrlMgr/48(MotAg0RawRes) -> [MotAg0RawRes]
  AR300FORDA_MotCtrlMgr/49(MotAg0SpiMecl) -> [MotAg0SpiMecl]
  AR300FORDA_MotCtrlMgr/50(MotAg0TurnCntrReg) -> [MotAg0TurnCntrReg]
  AR300FORDA_MotCtrlMgr/51(MotAg0VltgFltCnt) -> [MotAg0VltgFltCnt]
  AR300FORDA_MotCtrlMgr/52(MotAg0WarnReg) -> [MotAg0WarnReg]
  AR300FORDA_MotCtrlMgr/53(MotAg1ErrReg) -> [MotAg1ErrReg]
  AR300FORDA_MotCtrlMgr/54(MotAg1Mecl) -> [MotAg1Mecl]
  AR300FORDA_MotCtrlMgr/55(MotAg1MeclRollgCntr) -> [MotAg1MeclRollgCntr]
  AR300FORDA_MotCtrlMgr/56(MotAg1ParFltCnt) -> [MotAg1ParFltCnt]
  AR300FORDA_MotCtrlMgr/57(MotAg1RawMecl) -> [MotAg1RawMecl]
  AR300FORDA_MotCtrlMgr/58(MotAg1RawRes) -> [MotAg1RawRes]
  AR300FORDA_MotCtrlMgr/59(MotAg1SpiMecl) -> [MotAg1SpiMecl]
  AR300FORDA_MotCtrlMgr/60(MotAg1TurnCntrReg) -> [MotAg1TurnCntrReg]
  AR300FORDA_MotCtrlMgr/61(MotAg1VltgFltCnt) -> [MotAg1VltgFltCnt]
  AR300FORDA_MotCtrlMgr/62(MotAg1WarnReg) -> [MotAg1WarnReg]
  AR300FORDA_MotCtrlMgr/63(MotAg3Mecl) -> [MotAg3Mecl]
  AR300FORDA_MotCtrlMgr/64(MotAg4Mecl) -> [MotAg4Mecl]
  AR300FORDA_MotCtrlMgr/65(MotAg5Cos) -> [MotAg5Cos]
  AR300FORDA_MotCtrlMgr/66(MotAg5MeasTi) -> [MotAg5MeasTi]
  AR300FORDA_MotCtrlMgr/67(MotAg5Mecl) -> [MotAg5Mecl]
  AR300FORDA_MotCtrlMgr/68(MotAg5RawMecl) -> [MotAg5RawMecl]
  AR300FORDA_MotCtrlMgr/69(MotAg5Sin) -> [MotAg5Sin]
  AR300FORDA_MotCtrlMgr/70(MotAg6Cos) -> [MotAg6Cos]
  AR300FORDA_MotCtrlMgr/71(MotAg6MeasTi) -> [MotAg6MeasTi]
  AR300FORDA_MotCtrlMgr/72(MotAg6Mecl) -> [MotAg6Mecl]
  AR300FORDA_MotCtrlMgr/73(MotAg6RawMecl) -> [MotAg6RawMecl]
  AR300FORDA_MotCtrlMgr/74(MotAg6Sin) -> [MotAg6Sin]
  AR300FORDA_MotCtrlMgr/75(MotAgBuf) -> [MotAgBuf]
  AR300FORDA_MotCtrlMgr/76(MotAgBufIdx) -> [MotAgBufIdx]
  AR300FORDA_MotCtrlMgr/77(MotAgBuf_SigOut) -> [MotAgBuf_SigOut]
  AR300FORDA_MotCtrlMgr/78(MotAgCumvAlgndMrfRev) -> [MotAgCumvAlgndMrfRev]
  AR300FORDA_MotCtrlMgr/79(MotAgCumvInid) -> [MotAgCumvInid]
  AR300FORDA_MotCtrlMgr/80(MotAgElec) -> [MotAgElec]
  AR300FORDA_MotCtrlMgr/81(MotAgMeasTi) -> [MotAgMeasTi]
  AR300FORDA_MotCtrlMgr/82(MotAgMecl) -> [MotAgMecl]
  AR300FORDA_MotCtrlMgr/83(MotAgTiBuf) -> [MotAgTiBuf]
  AR300FORDA_MotCtrlMgr/84(MotAgTiBuf_SigOut) -> [MotAgTiBuf_SigOut]
  AR300FORDA_MotCtrlMgr/85(MotBackEmfVltg) -> AR300FORDA_MotCtrlMgr_MotBackEmfVltg/1
  AR300FORDA_MotCtrlMgr/86(MotCurr) -> [MotCurr]
  AR300FORDA_MotCtrlMgr/87(MotCurrAdcPeakA) -> [MotCurrAdcPeakA]
  AR300FORDA_MotCtrlMgr/88(MotCurrAdcPeakB) -> [MotCurrAdcPeakB]
  AR300FORDA_MotCtrlMgr/89(MotCurrAdcPeakC) -> [MotCurrAdcPeakC]
  AR300FORDA_MotCtrlMgr/90(MotCurrAdcPeakD) -> [MotCurrAdcPeakD]
  AR300FORDA_MotCtrlMgr/91(MotCurrAdcPeakE) -> [MotCurrAdcPeakE]
  AR300FORDA_MotCtrlMgr/92(MotCurrAdcPeakF) -> [MotCurrAdcPeakF]
  AR300FORDA_MotCtrlMgr/93(MotCurrAdcVlyA) -> [MotCurrAdcVlyA]
  AR300FORDA_MotCtrlMgr/94(MotCurrAdcVlyB) -> [MotCurrAdcVlyB]
  AR300FORDA_MotCtrlMgr/95(MotCurrAdcVlyC) -> [MotCurrAdcVlyC]
  AR300FORDA_MotCtrlMgr/96(MotCurrAdcVlyD) -> [MotCurrAdcVlyD]
  AR300FORDA_MotCtrlMgr/97(MotCurrAdcVlyE) -> [MotCurrAdcVlyE]
  AR300FORDA_MotCtrlMgr/98(MotCurrAdcVlyF) -> [MotCurrAdcVlyF]
  AR300FORDA_MotCtrlMgr/99(MotCurrCorrdA) -> [MotCurrCorrdA]
  AR300FORDA_MotCtrlMgr/100(MotCurrCorrdB) -> [MotCurrCorrdB]
  AR300FORDA_MotCtrlMgr/101(MotCurrCorrdC) -> [MotCurrCorrdC]
  AR300FORDA_MotCtrlMgr/102(MotCurrCorrdD) -> [MotCurrCorrdD]
  AR300FORDA_MotCtrlMgr/103(MotCurrCorrdE) -> [MotCurrCorrdE]
  AR300FORDA_MotCtrlMgr/104(MotCurrCorrdF) -> [MotCurrCorrdF]
  AR300FORDA_MotCtrlMgr/105(MotCurrDax) -> [MotCurrDax]
  AR300FORDA_MotCtrlMgr/106(MotCurrQax) -> [MotCurrQax]
  AR300FORDA_MotCtrlMgr/107(MotCurrQaxCmdFinal) -> [MotCurrQaxCmdFinal]
  AR300FORDA_MotCtrlMgr/108(MotCurrQaxCoggCmd) -> [MotCurrQaxCoggCmd]
  AR300FORDA_MotCtrlMgr/109(MotCurrQaxRplCmd) -> [MotCurrQaxRplCmd]
  AR300FORDA_MotCtrlMgr/110(MotCurrQlfr1) -> AR300FORDA_MotCtrlMgr_MotCurrQlfr1/1
  AR300FORDA_MotCtrlMgr/111(MotCurrQlfr2) -> [MotCurrQlfr2]
  AR300FORDA_MotCtrlMgr/112(MotCurrRollgCntr1) -> [MotCurrRollgCntr1]
  AR300FORDA_MotCtrlMgr/113(MotCurrRollgCntr2) -> [MotCurrRollgCntr2]
  AR300FORDA_MotCtrlMgr/114(MotCurrSnsrOffs1) -> [MotCurrSnsrOffs1]
  AR300FORDA_MotCtrlMgr/115(MotCurrSnsrOffs2) -> [MotCurrSnsrOffs2]
  AR300FORDA_MotCtrlMgr/116(MotInduDaxEstimdIvs) -> AR300FORDA_MotCtrlMgr_MotInduDaxEstimdIvs/1
  AR300FORDA_MotCtrlMgr/117(MotInduQaxEstimdIvs) -> AR300FORDA_MotCtrlMgr_MotInduQaxEstimdIvs/1
  AR300FORDA_MotCtrlMgr/118(MotModlnIdx) -> [MotModlnIdx]
  AR300FORDA_MotCtrlMgr/119(MotPhaAdv) -> [MotPhaAdv]
  AR300FORDA_MotCtrlMgr/120(MotVltg) -> [MotVltg]
  AR300FORDA_MotCtrlMgr/121(MotVltgCmdPolarity) -> [MotVltgCmdPolarity]
  AR300FORDA_MotCtrlMgr/122(MotVltgDax) -> [MotVltgDax]
  AR300FORDA_MotCtrlMgr/123(MotVltgDaxFild) -> [MotVltgDaxFild]
  AR300FORDA_MotCtrlMgr/124(MotVltgQax) -> [MotVltgQax]
  AR300FORDA_MotCtrlMgr/125(MotVltgQaxFild) -> [MotVltgQaxFild]
  AR300FORDA_MotCtrlMgr/126(Ntc5DErrCnt) -> [Ntc5DErrCnt]
  AR300FORDA_MotCtrlMgr/127(Ntc6DErrCnt) -> [Ntc6DErrCnt]
  AR300FORDA_MotCtrlMgr/128(PhaOnTiA) -> [PhaOnTiA]
  AR300FORDA_MotCtrlMgr/129(PhaOnTiB) -> [PhaOnTiB]
  AR300FORDA_MotCtrlMgr/130(PhaOnTiC) -> [PhaOnTiC]
  AR300FORDA_MotCtrlMgr/131(PhaOnTiSumA) -> [PhaOnTiSumA]
  AR300FORDA_MotCtrlMgr/132(PhaOnTiSumB) -> [PhaOnTiSumB]
  AR300FORDA_MotCtrlMgr/133(PhaOnTiSumC) -> [PhaOnTiSumC]
  AR300FORDA_MotCtrlMgr/134(PwmPerd) -> [PwmPerd]
  AR300FORDA_MotCtrlMgr/135(RegOutpCSIH1RRA) -> [RegOutpCSIH1RRA]
  AR300FORDA_MotCtrlMgr/136(SampleRdyFlgOutp) -> [SampleRdyFlgOutp]
  AR300FORDA_MotCtrlMgr/137(SlowLoopCntr) -> [SlowLoopCntr]
  AR300FORDA_MotCtrlMgr/138(SwCalEna) -> [SwCalEna]
  AR300FORDA_MotCtrlMgr/139(SwCalModlnIdx) -> [SwCalModlnIdx]
  AR300FORDA_MotCtrlMgr/140(SwCalPosnIdx) -> [SwCalPosnIdx]
  AR300FORDA_MotCtrlMgr/141(TSG31CMP0E) -> [TSG31CMP0E]
  AR300FORDA_MotCtrlMgr/142(TSG31CMP12E) -> [TSG31CMP12E]
  AR300FORDA_MotCtrlMgr/143(TSG31CMPUE) -> [TSG31CMPUE]
  AR300FORDA_MotCtrlMgr/144(TSG31CMPVE) -> [TSG31CMPVE]
  AR300FORDA_MotCtrlMgr/145(TSG31CMPWE) -> [TSG31CMPWE]
  AR300FORDA_MotCtrlMgr/146(TSG31DCMP0E) -> [TSG31DCMP0E]
  AR300FORDA_MotCtrlMgr/147(MotCtrlAdc0RawRes) -> AR300FORDA_MotCtrlMgr_MotCtrlAdc0RawRes/1
  AR300FORDA_MotCtrlMgr/148(MotCtrlAdc0ScanGroup2Ref0) -> AR300FORDA_MotCtrlMgr_MotCtrlAdc0ScanGroup2Ref0/1
  AR300FORDA_MotCtrlMgr/149(MotCtrlAdc0ScanGroup2Ref1) -> AR300FORDA_MotCtrlMgr_MotCtrlAdc0ScanGroup2Ref1/1
  AR300FORDA_MotCtrlMgr/150(MotCtrlAdc0ScanGroup3Ref0) -> AR300FORDA_MotCtrlMgr_MotCtrlAdc0ScanGroup3Ref0/1
  AR300FORDA_MotCtrlMgr/151(MotCtrlAdc0ScanGroup3Ref1) -> AR300FORDA_MotCtrlMgr_MotCtrlAdc0ScanGroup3Ref1/1
  AR300FORDA_MotCtrlMgr/152(MotCtrlAdc1RawRes) -> AR300FORDA_MotCtrlMgr_MotCtrlAdc1RawRes/1
  AR300FORDA_MotCtrlMgr/153(MotCtrlAdcDiagcEndPtrOutp) -> [MotCtrlAdcDiagcEndPtrOutp]
  AR300FORDA_MotCtrlMgr/154(MotCtrlAdcDiagcStrtPtrOutp) -> [MotCtrlAdcDiagcStrtPtrOutp]
  AR300FORDA_MotCtrlMgr/155(MotCtrlBattRtnCurrAdc) -> [MotCtrlBattRtnCurrAdc]
  AR300FORDA_MotCtrlMgr/156(MotCtrlBrdgVltg) -> [MotCtrlBrdgVltg]
  AR300FORDA_MotCtrlMgr/157(MotCtrlCtrlrTFild) -> [MotCtrlCtrlrTFild]
  AR300FORDA_MotCtrlMgr/158(MotCtrlCurrMeasCorrlnSts) -> [MotCtrlCurrMeasCorrlnSts]
  AR300FORDA_MotCtrlMgr/159(MotCtrlCurrMeasLoaMtgtnEna) -> [MotCtrlCurrMeasLoaMtgtnEna]
  AR300FORDA_MotCtrlMgr/160(MotCtrlCurrMeasMotAgCorrd) -> AR300FORDA_MotCtrlMgr_MotCtrlCurrMeasMotAgCorrd/1
  AR300FORDA_MotCtrlMgr/161(MotCtrlCurrMeasWrmIninTestCmpl) -> [MotCtrlCurrMeasWrmIninTestCmpl]
  AR300FORDA_MotCtrlMgr/162(MotCtrlDiagcStsIvtr1Inactv) -> [MotCtrlDiagcStsIvtr1Inactv]
  AR300FORDA_MotCtrlMgr/163(MotCtrlDiagcStsIvtr2Inactv) -> [MotCtrlDiagcStsIvtr2Inactv]
  AR300FORDA_MotCtrlMgr/164(MotCtrlDualEcuMotCtrlMtgtnEna) -> [MotCtrlDualEcuMotCtrlMtgtnEna]
  AR300FORDA_MotCtrlMgr/165(MotCtrlEcuTFild) -> [MotCtrlEcuTFild]
  AR300FORDA_MotCtrlMgr/166(MotCtrlHwTq4Raw) -> [MotCtrlHwTq4Raw]
  AR300FORDA_MotCtrlMgr/167(MotCtrlHwTq4RawFastAdc) -> [MotCtrlHwTq4RawFastAdc]
  AR300FORDA_MotCtrlMgr/168(MotCtrlHwTq5Raw) -> [MotCtrlHwTq5Raw]
  AR300FORDA_MotCtrlMgr/169(MotCtrlHwTq5RawFastAdc) -> [MotCtrlHwTq5RawFastAdc]
  AR300FORDA_MotCtrlMgr/170(MotCtrlIvtrFetFltPha) -> [MotCtrlIvtrFetFltPha]
  AR300FORDA_MotCtrlMgr/171(MotCtrlIvtrFetFltTyp) -> [MotCtrlIvtrFetFltTyp]
  AR300FORDA_MotCtrlMgr/172(MotCtrlIvtrLoaMtgtnEna) -> [MotCtrlIvtrLoaMtgtnEna]
  AR300FORDA_MotCtrlMgr/173(MotCtrlLoopCntr2MilliSec) -> [MotCtrlLoopCntr2MilliSec]
  AR300FORDA_MotCtrlMgr/174(MotCtrlMfgEnaSt) -> [MotCtrlMfgEnaSt]
  AR300FORDA_MotCtrlMgr/175(MotCtrlMotAg0ABIFaild) -> [MotCtrlMotAg0ABIFaild]
  AR300FORDA_MotCtrlMgr/176(MotCtrlMotAg0Offs) -> [MotCtrlMotAg0Offs]
  AR300FORDA_MotCtrlMgr/177(MotCtrlMotAg0QepFaild) -> [MotCtrlMotAg0QepFaild]
  AR300FORDA_MotCtrlMgr/178(MotCtrlMotAg0RawRes) -> [MotCtrlMotAg0RawRes]
  AR300FORDA_MotCtrlMgr/179(MotCtrlMotAg1ABIFaild) -> [MotCtrlMotAg1ABIFaild]
  AR300FORDA_MotCtrlMgr/180(MotCtrlMotAg1Offs) -> [MotCtrlMotAg1Offs]
  AR300FORDA_MotCtrlMgr/181(MotCtrlMotAg1QepFaild) -> [MotCtrlMotAg1QepFaild]
  AR300FORDA_MotCtrlMgr/182(MotCtrlMotAg1RawRes) -> [MotCtrlMotAg1RawRes]
  AR300FORDA_MotCtrlMgr/183(MotCtrlMotAg2Cos) -> [MotCtrlMotAg2Cos]
  AR300FORDA_MotCtrlMgr/184(MotCtrlMotAg2CosAdcFaild) -> [MotCtrlMotAg2CosAdcFaild]
  AR300FORDA_MotCtrlMgr/185(MotCtrlMotAg2Sin) -> [MotCtrlMotAg2Sin]
  AR300FORDA_MotCtrlMgr/186(MotCtrlMotAg2SinAdcFaild) -> [MotCtrlMotAg2SinAdcFaild]
  AR300FORDA_MotCtrlMgr/187(MotCtrlMotAg5Cos) -> AR300FORDA_MotCtrlMgr_MotCtrlMotAg5Cos/1
  AR300FORDA_MotCtrlMgr/188(MotCtrlMotAg5CosAdcFaild) -> [MotCtrlMotAg5CosAdcFaild]
  AR300FORDA_MotCtrlMgr/189(MotCtrlMotAg5CosRtAmpRecpr) -> [MotCtrlMotAg5CosRtAmpRecpr]
  AR300FORDA_MotCtrlMgr/190(MotCtrlMotAg5CosRtAmpRecpr1) -> [MotCtrlMotAg5CosRtAmpRecpr1]
  AR300FORDA_MotCtrlMgr/191(MotCtrlMotAg5CosRtOffs) -> [MotCtrlMotAg5CosRtOffs]
  AR300FORDA_MotCtrlMgr/192(MotCtrlMotAg5CosRtOffs1) -> [MotCtrlMotAg5CosRtOffs1]
  AR300FORDA_MotCtrlMgr/193(MotCtrlMotAg5Polarity) -> [MotCtrlMotAg5Polarity]
  AR300FORDA_MotCtrlMgr/194(MotCtrlMotAg5Sin) -> AR300FORDA_MotCtrlMgr_MotCtrlMotAg5Sin/1
  AR300FORDA_MotCtrlMgr/195(MotCtrlMotAg5SinAdcFaild) -> [MotCtrlMotAg5SinAdcFaild]
  AR300FORDA_MotCtrlMgr/196(MotCtrlMotAg5SinRtAmpRecpr) -> [MotCtrlMotAg5SinRtAmpRecpr]
  AR300FORDA_MotCtrlMgr/197(MotCtrlMotAg5SinRtAmpRecpr1) -> [MotCtrlMotAg5SinRtAmpRecpr1]
  AR300FORDA_MotCtrlMgr/198(MotCtrlMotAg5SinRtOffs) -> [MotCtrlMotAg5SinRtOffs]
  AR300FORDA_MotCtrlMgr/199(MotCtrlMotAg5SinRtOffs1) -> [MotCtrlMotAg5SinRtOffs1]
  AR300FORDA_MotCtrlMgr/200(MotCtrlMotAg6Cos) -> AR300FORDA_MotCtrlMgr_MotCtrlMotAg6Cos/1
  AR300FORDA_MotCtrlMgr/201(MotCtrlMotAg6CosAdcFaild) -> [MotCtrlMotAg6CosAdcFaild]
  AR300FORDA_MotCtrlMgr/202(MotCtrlMotAg6CosRtAmpRecpr) -> [MotCtrlMotAg6CosRtAmpRecpr]
  AR300FORDA_MotCtrlMgr/203(MotCtrlMotAg6CosRtAmpRecpr1) -> [MotCtrlMotAg6CosRtAmpRecpr1]
  AR300FORDA_MotCtrlMgr/204(MotCtrlMotAg6CosRtOffs) -> [MotCtrlMotAg6CosRtOffs]
  AR300FORDA_MotCtrlMgr/205(MotCtrlMotAg6CosRtOffs1) -> [MotCtrlMotAg6CosRtOffs1]
  AR300FORDA_MotCtrlMgr/206(MotCtrlMotAg6Polarity) -> [MotCtrlMotAg6Polarity]
  AR300FORDA_MotCtrlMgr/207(MotCtrlMotAg6Sin) -> AR300FORDA_MotCtrlMgr_MotCtrlMotAg6Sin/1
  AR300FORDA_MotCtrlMgr/208(MotCtrlMotAg6SinAdcFaild) -> [MotCtrlMotAg6SinAdcFaild]
  AR300FORDA_MotCtrlMgr/209(MotCtrlMotAg6SinRtAmpRecpr) -> [MotCtrlMotAg6SinRtAmpRecpr]
  AR300FORDA_MotCtrlMgr/210(MotCtrlMotAg6SinRtAmpRecpr1) -> [MotCtrlMotAg6SinRtAmpRecpr1]
  AR300FORDA_MotCtrlMgr/211(MotCtrlMotAg6SinRtOffs) -> [MotCtrlMotAg6SinRtOffs]
  AR300FORDA_MotCtrlMgr/212(MotCtrlMotAg6SinRtOffs1) -> [MotCtrlMotAg6SinRtOffs1]
  AR300FORDA_MotCtrlMgr/213(MotCtrlMotAgAMecl) -> [MotCtrlMotAgAMecl]
  AR300FORDA_MotCtrlMgr/214(MotCtrlMotAgAMeclQlfr) -> [MotCtrlMotAgAMeclQlfr]
  AR300FORDA_MotCtrlMgr/215(MotCtrlMotAgAMeclRollgCntr) -> [MotCtrlMotAgAMeclRollgCntr]
  AR300FORDA_MotCtrlMgr/216(MotCtrlMotAgBMecl) -> [MotCtrlMotAgBMecl]
  AR300FORDA_MotCtrlMgr/217(MotCtrlMotAgBMeclQlfr) -> [MotCtrlMotAgBMeclQlfr]
  AR300FORDA_MotCtrlMgr/218(MotCtrlMotAgBMeclRollgCntr) -> [MotCtrlMotAgBMeclRollgCntr]
  AR300FORDA_MotCtrlMgr/219(MotCtrlMotAgBuf) -> [MotCtrlMotAgBuf]
  AR300FORDA_MotCtrlMgr/220(MotCtrlMotAgBuf_SigIn) -> [MotCtrlMotAgBuf_SigIn]
  AR300FORDA_MotCtrlMgr/221(MotCtrlMotAgCorrd) -> [MotCtrlMotAgCorrd]
  AR300FORDA_MotCtrlMgr/222(MotCtrlMotAgElec) -> AR300FORDA_MotCtrlMgr_MotCtrlMotAgElec/1
  AR300FORDA_MotCtrlMgr/223(MotCtrlMotAgElecDly) -> [MotCtrlMotAgElecDly]
  AR300FORDA_MotCtrlMgr/224(MotCtrlMotAgElecDlyRpl) -> [MotCtrlMotAgElecDlyRpl]
  AR300FORDA_MotCtrlMgr/225(MotCtrlMotAgMeasTi) -> AR300FORDA_MotCtrlMgr_MotCtrlMotAgMeasTi/1
  AR300FORDA_MotCtrlMgr/226(MotCtrlMotAgMecl) -> [MotCtrlMotAgMecl]
  AR300FORDA_MotCtrlMgr/227(MotCtrlMotAgMecl0Polarity) -> [MotCtrlMotAgMecl0Polarity]
  AR300FORDA_MotCtrlMgr/228(MotCtrlMotAgMecl1Polarity) -> [MotCtrlMotAgMecl1Polarity]
  AR300FORDA_MotCtrlMgr/229(MotCtrlMotAgMeclCorrlnSt) -> [MotCtrlMotAgMeclCorrlnSt]
  AR300FORDA_MotCtrlMgr/230(MotCtrlMotAgMeclCorrlnSts) -> [MotCtrlMotAgMeclCorrlnSts]
  AR300FORDA_MotCtrlMgr/231(MotCtrlMotAgTiBuf) -> [MotCtrlMotAgTiBuf]
  AR300FORDA_MotCtrlMgr/232(MotCtrlMotAgTiBuf_SigIn) -> [MotCtrlMotAgTiBuf_SigIn]
  AR300FORDA_MotCtrlMgr/233(MotCtrlMotAndThermProtnLoaMod) -> [MotCtrlMotAndThermProtnLoaMod]
  AR300FORDA_MotCtrlMgr/234(MotCtrlMotBackEmfVltg) -> [MotCtrlMotBackEmfVltg]
  AR300FORDA_MotCtrlMgr/235(MotCtrlMotCurr) -> [MotCtrlMotCurr]
  AR300FORDA_MotCtrlMgr/236(MotCtrlMotCurrAdcVlyA) -> AR300FORDA_MotCtrlMgr_MotCtrlMotCurrAdcVlyA/1
  AR300FORDA_MotCtrlMgr/237(MotCtrlMotCurrAdcVlyAAdcFaild) -> [MotCtrlMotCurrAdcVlyAAdcFaild]
  AR300FORDA_MotCtrlMgr/238(MotCtrlMotCurrAdcVlyB) -> AR300FORDA_MotCtrlMgr_MotCtrlMotCurrAdcVlyB/1
  AR300FORDA_MotCtrlMgr/239(MotCtrlMotCurrAdcVlyBAdcFaild) -> [MotCtrlMotCurrAdcVlyBAdcFaild]
  AR300FORDA_MotCtrlMgr/240(MotCtrlMotCurrAdcVlyC) -> AR300FORDA_MotCtrlMgr_MotCtrlMotCurrAdcVlyC/1
  AR300FORDA_MotCtrlMgr/241(MotCtrlMotCurrAdcVlyCAdcFaild) -> [MotCtrlMotCurrAdcVlyCAdcFaild]
  AR300FORDA_MotCtrlMgr/242(MotCtrlMotCurrAdcVlyD) -> [MotCtrlMotCurrAdcVlyD]
  AR300FORDA_MotCtrlMgr/243(MotCtrlMotCurrAdcVlyDAdcFaild) -> [MotCtrlMotCurrAdcVlyDAdcFaild]
  AR300FORDA_MotCtrlMgr/244(MotCtrlMotCurrAdcVlyE) -> [MotCtrlMotCurrAdcVlyE]
  AR300FORDA_MotCtrlMgr/245(MotCtrlMotCurrAdcVlyEAdcFaild) -> [MotCtrlMotCurrAdcVlyEAdcFaild]
  AR300FORDA_MotCtrlMgr/246(MotCtrlMotCurrAdcVlyF) -> [MotCtrlMotCurrAdcVlyF]
  AR300FORDA_MotCtrlMgr/247(MotCtrlMotCurrAdcVlyFAdcFaild) -> [MotCtrlMotCurrAdcVlyFAdcFaild]
  AR300FORDA_MotCtrlMgr/248(MotCtrlMotCurrCmd) -> [MotCtrlMotCurrCmd]
  AR300FORDA_MotCtrlMgr/249(MotCtrlMotCurrCorrdA) -> [MotCtrlMotCurrCorrdA]
  AR300FORDA_MotCtrlMgr/250(MotCtrlMotCurrCorrdB) -> [MotCtrlMotCurrCorrdB]
  AR300FORDA_MotCtrlMgr/251(MotCtrlMotCurrCorrdC) -> [MotCtrlMotCurrCorrdC]
  AR300FORDA_MotCtrlMgr/252(MotCtrlMotCurrCorrdD) -> [MotCtrlMotCurrCorrdD]
  AR300FORDA_MotCtrlMgr/253(MotCtrlMotCurrCorrdE) -> [MotCtrlMotCurrCorrdE]
  AR300FORDA_MotCtrlMgr/254(MotCtrlMotCurrCorrdF) -> [MotCtrlMotCurrCorrdF]
  AR300FORDA_MotCtrlMgr/255(MotCtrlMotCurrDax) -> AR300FORDA_MotCtrlMgr_MotCtrlMotCurrDax/1
  AR300FORDA_MotCtrlMgr/256(MotCtrlMotCurrDaxCmd) -> [MotCtrlMotCurrDaxCmd]
  AR300FORDA_MotCtrlMgr/257(MotCtrlMotCurrDaxMax) -> [MotCtrlMotCurrDaxMax]
  AR300FORDA_MotCtrlMgr/258(MotCtrlMotCurrEolCalSt) -> [MotCtrlMotCurrEolCalSt]
  AR300FORDA_MotCtrlMgr/259(MotCtrlMotCurrLoaMtgtnEna) -> [MotCtrlMotCurrLoaMtgtnEna]
  AR300FORDA_MotCtrlMgr/260(MotCtrlMotCurrQax) -> AR300FORDA_MotCtrlMgr_MotCtrlMotCurrQax/1
  AR300FORDA_MotCtrlMgr/261(MotCtrlMotCurrQaxCmd) -> [MotCtrlMotCurrQaxCmd]
  AR300FORDA_MotCtrlMgr/262(MotCtrlMotCurrQaxCoggCmd) -> AR300FORDA_MotCtrlMgr_MotCtrlMotCurrQaxCoggCmd/1
  AR300FORDA_MotCtrlMgr/263(MotCtrlMotCurrQaxRplCmd) -> AR300FORDA_MotCtrlMgr_MotCtrlMotCurrQaxRplCmd/1
  AR300FORDA_MotCtrlMgr/264(MotCtrlMotCurrQaxToMotTqGain) -> [MotCtrlMotCurrQaxToMotTqGain]
  AR300FORDA_MotCtrlMgr/265(MotCtrlMotCurrQlfr1) -> [MotCtrlMotCurrQlfr1]
  AR300FORDA_MotCtrlMgr/266(MotCtrlMotCurrQlfr2) -> [MotCtrlMotCurrQlfr2]
  AR300FORDA_MotCtrlMgr/267(MotCtrlMotCurrRollgCntr1) -> [MotCtrlMotCurrRollgCntr1]
  AR300FORDA_MotCtrlMgr/268(MotCtrlMotCurrRollgCntr2) -> [MotCtrlMotCurrRollgCntr2]
  AR300FORDA_MotCtrlMgr/269(MotCtrlMotDampgDax) -> [MotCtrlMotDampgDax]
  AR300FORDA_MotCtrlMgr/270(MotCtrlMotDampgQax) -> [MotCtrlMotDampgQax]
  AR300FORDA_MotCtrlMgr/271(MotCtrlMotElecMeclPolarity) -> [MotCtrlMotElecMeclPolarity]
  AR300FORDA_MotCtrlMgr/272(MotCtrlMotInduDaxEstimdIvs) -> [MotCtrlMotInduDaxEstimdIvs]
  AR300FORDA_MotCtrlMgr/273(MotCtrlMotInduQaxEstimdIvs) -> [MotCtrlMotInduQaxEstimdIvs]
  AR300FORDA_MotCtrlMgr/274(MotCtrlMotIntglGain) -> [MotCtrlMotIntglGain]
  AR300FORDA_MotCtrlMgr/275(MotCtrlMotIntglGainDax) -> [MotCtrlMotIntglGainDax]
  AR300FORDA_MotCtrlMgr/276(MotCtrlMotIntglGainQax) -> [MotCtrlMotIntglGainQax]
  AR300FORDA_MotCtrlMgr/277(MotCtrlMotModlnIdx) -> AR300FORDA_MotCtrlMgr_MotCtrlMotModlnIdx/1
  AR300FORDA_MotCtrlMgr/278(MotCtrlMotPhaAdv) -> AR300FORDA_MotCtrlMgr_MotCtrlMotPhaAdv/1
  AR300FORDA_MotCtrlMgr/279(MotCtrlMotPropGain) -> [MotCtrlMotPropGain]
  AR300FORDA_MotCtrlMgr/280(MotCtrlMotPropGainDax) -> [MotCtrlMotPropGainDax]
  AR300FORDA_MotCtrlMgr/281(MotCtrlMotPropGainQax) -> [MotCtrlMotPropGainQax]
  AR300FORDA_MotCtrlMgr/282(MotCtrlMotREstimd) -> [MotCtrlMotREstimd]
  AR300FORDA_MotCtrlMgr/283(MotCtrlMotReacncDax) -> [MotCtrlMotReacncDax]
  AR300FORDA_MotCtrlMgr/284(MotCtrlMotReacncQax) -> [MotCtrlMotReacncQax]
  AR300FORDA_MotCtrlMgr/285(MotCtrlMotTqRplCoggOrder1Mgn) -> [MotCtrlMotTqRplCoggOrder1Mgn]
  AR300FORDA_MotCtrlMgr/286(MotCtrlMotTqRplCoggOrder1Pha) -> [MotCtrlMotTqRplCoggOrder1Pha]
  AR300FORDA_MotCtrlMgr/287(MotCtrlMotTqRplCoggOrder2Mgn) -> [MotCtrlMotTqRplCoggOrder2Mgn]
  AR300FORDA_MotCtrlMgr/288(MotCtrlMotTqRplCoggOrder2Pha) -> [MotCtrlMotTqRplCoggOrder2Pha]
  AR300FORDA_MotCtrlMgr/289(MotCtrlMotTqRplCoggOrder3Mgn) -> [MotCtrlMotTqRplCoggOrder3Mgn]
  AR300FORDA_MotCtrlMgr/290(MotCtrlMotTqRplCoggOrder3Pha) -> [MotCtrlMotTqRplCoggOrder3Pha]
  AR300FORDA_MotCtrlMgr/291(MotCtrlMotVelMrf) -> [MotCtrlMotVelMrf]
  AR300FORDA_MotCtrlMgr/292(MotCtrlMotVltgCmdPolarity) -> [MotCtrlMotVltgCmdPolarity]
  AR300FORDA_MotCtrlMgr/293(MotCtrlMotVltgDax) -> AR300FORDA_MotCtrlMgr_MotCtrlMotVltgDax/1
  AR300FORDA_MotCtrlMgr/294(MotCtrlMotVltgDaxFf) -> [MotCtrlMotVltgDaxFf]
  AR300FORDA_MotCtrlMgr/295(MotCtrlMotVltgQax) -> AR300FORDA_MotCtrlMgr_MotCtrlMotVltgQax/1
  AR300FORDA_MotCtrlMgr/296(MotCtrlMotVltgQaxFf) -> [MotCtrlMotVltgQaxFf]
  AR300FORDA_MotCtrlMgr/297(MotCtrlPhaDiscnctDiagcActv) -> [MotCtrlPhaDiscnctDiagcActv]
  AR300FORDA_MotCtrlMgr/298(MotCtrlPhaDiscnctDiagcPwmVect) -> [MotCtrlPhaDiscnctDiagcPwmVect]
  AR300FORDA_MotCtrlMgr/299(MotCtrlPhaOnTiA) -> AR300FORDA_MotCtrlMgr_MotCtrlPhaOnTiA/1
  AR300FORDA_MotCtrlMgr/300(MotCtrlPhaOnTiB) -> AR300FORDA_MotCtrlMgr_MotCtrlPhaOnTiB/1
  AR300FORDA_MotCtrlMgr/301(MotCtrlPhaOnTiC) -> AR300FORDA_MotCtrlMgr_MotCtrlPhaOnTiC/1
  AR300FORDA_MotCtrlMgr/302(MotCtrlPhaOnTiSumA) -> AR300FORDA_MotCtrlMgr_MotCtrlPhaOnTiSumA/1
  AR300FORDA_MotCtrlMgr/303(MotCtrlPhaOnTiSumB) -> AR300FORDA_MotCtrlMgr_MotCtrlPhaOnTiSumB/1
  AR300FORDA_MotCtrlMgr/304(MotCtrlPhaOnTiSumC) -> AR300FORDA_MotCtrlMgr_MotCtrlPhaOnTiSumC/1
  AR300FORDA_MotCtrlMgr/305(MotCtrlPwmPerd) -> AR300FORDA_MotCtrlMgr_MotCtrlPwmPerd/1
  AR300FORDA_MotCtrlMgr/306(MotCtrlSampleRdyFlgInp) -> [MotCtrlSampleRdyFlgInp]
  AR300FORDA_MotCtrlMgr/307(MotCtrlStrtUpSt) -> [MotCtrlStrtUpSt]
  AR300FORDA_MotCtrlMgr/308(MotCtrlSwCalEna) -> AR300FORDA_MotCtrlMgr_MotCtrlSwCalEna/1
  AR300FORDA_MotCtrlMgr/309(MotCtrlSwCalModlnIdx) -> AR300FORDA_MotCtrlMgr_MotCtrlSwCalModlnIdx/1
  AR300FORDA_MotCtrlMgr/310(MotCtrlSwCalPosnIdx) -> AR300FORDA_MotCtrlMgr_MotCtrlSwCalPosnIdx/1
  AR300FORDA_MotCtrlMgr/311(MotCtrlSysSt) -> [MotCtrlSysSt]
  AR300FORDA_MotCtrlMgr/312(MotCtrlTSG31CMPVE) -> [MotCtrlTSG31CMPVE]
  AR300FORDA_MotCtrlMgr/313(MotCtrlTSG31CMPWE) -> [MotCtrlTSG31CMPWE]
  AR300FORDA_MotCtrlMgr/314(MotCtrlTSG31DCMP0E) -> [MotCtrlTSG31DCMP0E]
  AR300FORDA_MotCtrlMgr/315(MotCtrlVehSpd) -> [MotCtrlVehSpd]
